simulink model "Prefeeded_Control"  (R2025a)
settings: Solver=VariableStepAuto  StartTime=0.0  StopTime=10.0  RelTol=1e-3
undefined symbols (not defined in the file or in its folder): B, J
settings Model: Creator=yurru  LastModifiedBy=yurru

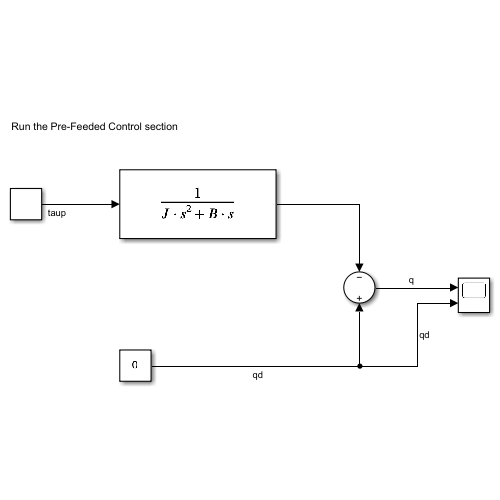
[thumbnail: Simulink's stored preview of the top-level diagram]
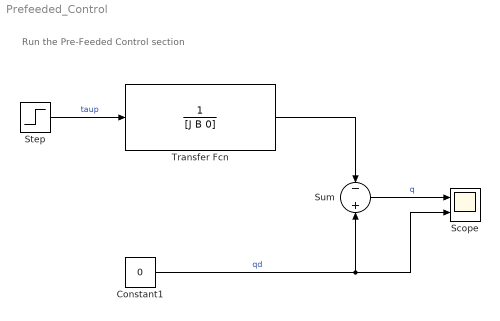
== system Prefeeded_Control ==
  note: Run the Pre-Feeded Control section
  Constant1 : Constant  Value=0
  Scope : Scope  NumInputPorts=2
      settings: ActiveDisplayYMinimum=-1.5799990485161415  ActiveDisplayYMaximum=0.1755554498351268
  Step : Step  SampleTime=0
  Sum : Sum  Inputs=-|+
  Transfer Fcn : TransferFcn  Denominator=[J B 0]
  wires:
  Constant1/1 -> Sum/2, Scope/2  "qd"
  Transfer Fcn/1 -> Sum/1
  Sum/1 -> Scope/1  "q"
  Step/1 -> Transfer Fcn/1  "taup"
